simulink model "foc_controller"  (R2023b)
settings: Solver=FixedStepDiscrete  StartTime=0.0  StopTime=0.01  FixedStep=Ts_ctrl  RelTol=1e-3
model workspace (MATLAB code in the model file):
  | % FOC controller parameters
  | % Placeholder values for structural modelling only; no tuning intended.
  | 
  | fs_ctrl = 5000.0;    % controller discrete update frequency [Hz] (placeholder)
  | Ts_ctrl = 1/fs_ctrl; % controller discrete update period [s] (placeholder)
  | 
  | Kp_id = 5;           % d-axis current-loop proportional gain (placeholder)
  | Ki_id = 100;         % d-axis current-loop integral gain (placeholder)
  | 
  | Kp_iq = 5;           % q-axis current-loop proportional gain (placeholder)
  | Ki_iq = 100;         % q-axis current-loop integral gain (placeholder)
  | 
  | Ld_comp = 2e-3;      % d-axis-related compensation coefficient (placeholder)
  | Lq_comp = 2e-3;      % q-axis-related compensation coefficient (placeholder)
  | psi_f_comp = 0.1;    % flux-related compensation coefficient (placeholder)
  | 
  | comp_d_sign = -1;    % d-axis compensation sign (placeholder)
  | comp_q_sign = 1;     % q-axis compensation sign (placeholder)
libraries: slpidlib x2
settings Model: Creator=hwma  LastModifiedBy=hwma

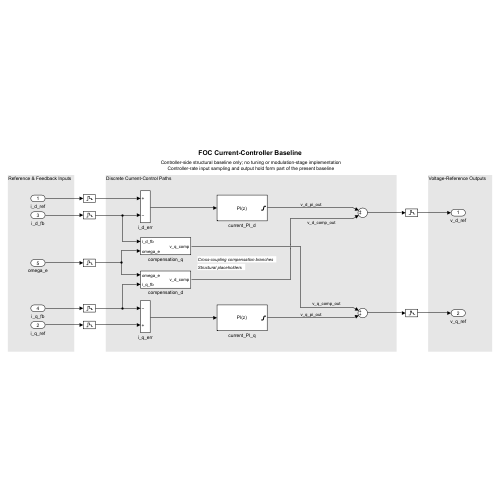
[thumbnail: Simulink's stored preview of the top-level diagram]
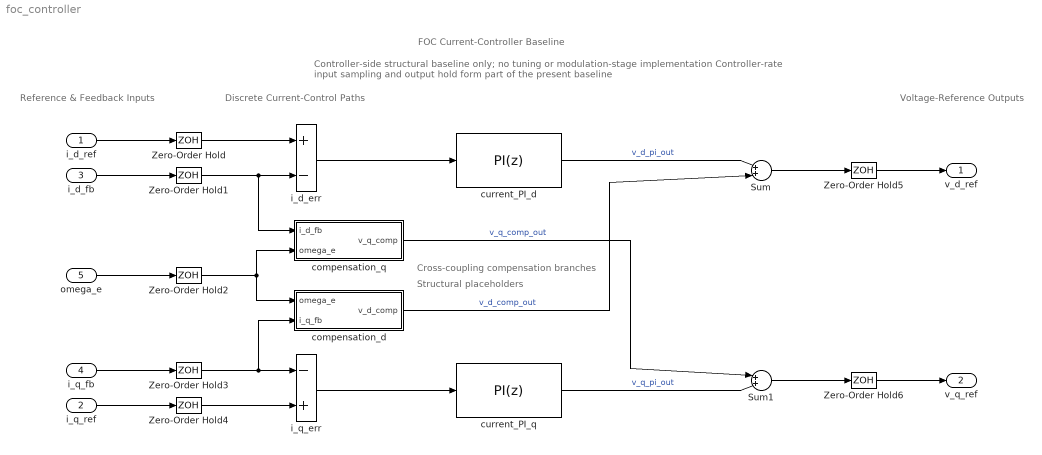
== system foc_controller ==
  note: Cross-coupling compensation branches
  note: Reference & Feedback Inputs
  note: Discrete Current-Control Paths
  note: Voltage-Reference Outputs
  note: Controller-side structural baseline only; no tuning or modulation-stage implementation Controller-rate input sampling and output hold form part of the present baseline
  note: FOC Current-Controller Baseline
  note: Structural placeholders
  i_d_ref : Inport
  i_q_ref : Inport  Port=2
  i_d_fb : Inport  Port=3
  i_q_fb : Inport  Port=4
  omega_e : Inport  Port=5
  Sum : Sum  Inputs=|++|
  Sum1 : Sum  Inputs=|++|
  Zero-Order Hold{,1..6} (7 alike) : ZeroOrderHold  SampleTime=Ts_ctrl
  compensation_d : Subsystem
  compensation_q : Subsystem
  current_PI_d : slpidlib/PID Controller  Controller=PI  Form=Parallel  TimeDomain=Discrete-time  UseExternalTs=off  SampleTime=Ts_ctrl  IntegratorMethod=Forward Euler  FilterMethod=Forward Euler  ControllerParametersSource=internal  P=Kp_id  I=Ki_id  UseKiTs=off  D=0  N=100  UseFilter=on  TunerSelectOption=Transfer Function Based (PID Tuner App)  InitialConditionSource=internal  InitialConditionForIntegrator=0  InitialConditionForFilter=0  DifferentiatorICPrevScaledInput=0  ExternalReset=none  TrackingMode=off  Kt=1  LimitOutput=on  SatLimitsSource=internal  UpperSaturationLimit=440  LowerSaturationLimit=-440  LinearizeAsGain=off  AntiWindupMode=none  Kb=1  LimitIntegrator=on  UpperIntegratorSaturationLimit=440  LowerIntegratorSaturationLimit=-440  POutMin=[]  POutMax=[]  IOutMin=[]  IOutMax=[]  DOutMin=[]  DOutMax=[]  NOutMin=[]  NOutMax=[]  SumOutMin=[]  SumOutMax=[]  SaturationOutMin=[]  SaturationOutMax=[]  PParamMin=[]  PParamMax=[]  IParamMin=[]  IParamMax=[]  DParamMin=[]  DParamMax=[]  NParamMin=[]  NParamMax=[]  KbParamMin=[]  KbParamMax=[]  KtParamMin=[]  KtParamMax=[]  KbOutMin=[]  KbOutMax=[]  KtOutMin=[]  KtOutMax=[]  IntegratorOutMin=[]  IntegratorOutMax=[]  FilterOutMin=[]  FilterOutMax=[]  SumI1OutMin=[]  SumI1OutMax=[]  SumI2OutMin=[]  SumI2OutMax=[]  SumI3OutMin=[]  SumI3OutMax=[]  SumI4OutMin=[]  SumI4OutMax=[]  SumDOutMin=[]  SumDOutMax=[]  DifferentiatorOutMin=[]  DifferentiatorOutMax=[]  FilterDiffOutCoefMin=[]  FilterDiffOutCoefMax=[]  ReciprocalOutMin=[]  ReciprocalOutMax=[]  SumDenOutMin=[]  SumDenOutMax=[]  SumNumOutMin=[]  SumNumOutMax=[]  DivideOutMin=[]  DivideOutMax=[]  UdiffTsProdOutMin=[]  UdiffTsProdOutMax=[]  NTsProdOutMin=[]  NTsProdOutMax=[]  UintegralTsProdOutMin=[]  UintegralTsProdOutMax=[]  UngainTsProdOutMin=[]  UngainTsProdOutMax=[]  ClampingZeroOutDataTypeStr=Inherit: Inherit via back propagation  ClampingZeroOutMin=[]  ClampingZeroOutMax=[]  FilterDenConstantOutDataTypeStr=Inherit: Inherit via back propagation  FilterDenConstantOutMin=[]  FilterDenConstantOutMax=[]  PCopyOutDataTypeStr=Inherit: Inherit via back propagation  PCopyOutMin=[]  PCopyOutMax=[]  NCopyOutDataTypeStr=Inherit: Inherit via back propagation  NCopyOutMin=[]  NCopyOutMax=[]  IntegratorContinuousStateAttributes=''  IntegratorStateMustResolveToSignalObject=off  IntegratorRTWStateStorageClass=Auto  FilterContinuousStateAttributes=''  FilterStateMustResolveToSignalObject=off  FilterRTWStateStorageClass=Auto  ParallelPVariant=InternalParameters  IdealPVariant=Disabled  IVariant=InternalParameters  DVariant=Disabled  IntegratorVariant=Discrete  SatVariant=Enabled  AWVariant=Passthrough  PCopyVariant=Disabled  TRVariant=Disabled  FdbkBlocksVariant=Forward  IdealPFdbkVariant=Disabled  SatFdbkVariant=Disabled  DerivativeFilterVariant=Disabled  NVariant=Disabled  NCopyVariant=Disabled_SignalSpec  FilterICVariant=Disabled  IntegratorICVariant=InternalICs  ExternalResetVariant=Disabled  TRSumVariant=Passthrough  SumFdbkVariant=Disabled  SumVariant=Sum_PI  TsampFilterVariant=InternalTs  TsampNgainVariant=Passthrough  TsampIntegralVariant=Disabled_SignalSpec  ExternalSaturationOutDataTypeStr=Inherit: Same as second input
      settings: LibrarySourceBlock=simulink/Discrete/Discrete PID Controller
  current_PI_q : slpidlib/PID Controller  Controller=PI  Form=Parallel  TimeDomain=Discrete-time  UseExternalTs=off  SampleTime=Ts_ctrl  IntegratorMethod=Forward Euler  FilterMethod=Forward Euler  ControllerParametersSource=internal  P=Kp_iq  I=Ki_iq  UseKiTs=off  D=0  N=100  UseFilter=on  TunerSelectOption=Transfer Function Based (PID Tuner App)  InitialConditionSource=internal  InitialConditionForIntegrator=0  InitialConditionForFilter=0  DifferentiatorICPrevScaledInput=0  ExternalReset=none  TrackingMode=off  Kt=1  LimitOutput=on  SatLimitsSource=internal  UpperSaturationLimit=440  LowerSaturationLimit=-440  LinearizeAsGain=off  AntiWindupMode=none  Kb=1  LimitIntegrator=on  UpperIntegratorSaturationLimit=440  LowerIntegratorSaturationLimit=-440  POutMin=[]  POutMax=[]  IOutMin=[]  IOutMax=[]  DOutMin=[]  DOutMax=[]  NOutMin=[]  NOutMax=[]  SumOutMin=[]  SumOutMax=[]  SaturationOutMin=[]  SaturationOutMax=[]  PParamMin=[]  PParamMax=[]  IParamMin=[]  IParamMax=[]  DParamMin=[]  DParamMax=[]  NParamMin=[]  NParamMax=[]  KbParamMin=[]  KbParamMax=[]  KtParamMin=[]  KtParamMax=[]  KbOutMin=[]  KbOutMax=[]  KtOutMin=[]  KtOutMax=[]  IntegratorOutMin=[]  IntegratorOutMax=[]  FilterOutMin=[]  FilterOutMax=[]  SumI1OutMin=[]  SumI1OutMax=[]  SumI2OutMin=[]  SumI2OutMax=[]  SumI3OutMin=[]  SumI3OutMax=[]  SumI4OutMin=[]  SumI4OutMax=[]  SumDOutMin=[]  SumDOutMax=[]  DifferentiatorOutMin=[]  DifferentiatorOutMax=[]  FilterDiffOutCoefMin=[]  FilterDiffOutCoefMax=[]  ReciprocalOutMin=[]  ReciprocalOutMax=[]  SumDenOutMin=[]  SumDenOutMax=[]  SumNumOutMin=[]  SumNumOutMax=[]  DivideOutMin=[]  DivideOutMax=[]  UdiffTsProdOutMin=[]  UdiffTsProdOutMax=[]  NTsProdOutMin=[]  NTsProdOutMax=[]  UintegralTsProdOutMin=[]  UintegralTsProdOutMax=[]  UngainTsProdOutMin=[]  UngainTsProdOutMax=[]  ClampingZeroOutDataTypeStr=Inherit: Inherit via back propagation  ClampingZeroOutMin=[]  ClampingZeroOutMax=[]  FilterDenConstantOutDataTypeStr=Inherit: Inherit via back propagation  FilterDenConstantOutMin=[]  FilterDenConstantOutMax=[]  PCopyOutDataTypeStr=Inherit: Inherit via back propagation  PCopyOutMin=[]  PCopyOutMax=[]  NCopyOutDataTypeStr=Inherit: Inherit via back propagation  NCopyOutMin=[]  NCopyOutMax=[]  IntegratorContinuousStateAttributes=''  IntegratorStateMustResolveToSignalObject=off  IntegratorRTWStateStorageClass=Auto  FilterContinuousStateAttributes=''  FilterStateMustResolveToSignalObject=off  FilterRTWStateStorageClass=Auto  ParallelPVariant=InternalParameters  IdealPVariant=Disabled  IVariant=InternalParameters  DVariant=Disabled  IntegratorVariant=Discrete  SatVariant=Enabled  AWVariant=Passthrough  PCopyVariant=Disabled  TRVariant=Disabled  FdbkBlocksVariant=Forward  IdealPFdbkVariant=Disabled  SatFdbkVariant=Disabled  DerivativeFilterVariant=Disabled  NVariant=Disabled  NCopyVariant=Disabled_SignalSpec  FilterICVariant=Disabled  IntegratorICVariant=InternalICs  ExternalResetVariant=Disabled  TRSumVariant=Passthrough  SumFdbkVariant=Disabled  SumVariant=Sum_PI  TsampFilterVariant=InternalTs  TsampNgainVariant=Passthrough  TsampIntegralVariant=Disabled_SignalSpec  ExternalSaturationOutDataTypeStr=Inherit: Same as second input
      settings: LibrarySourceBlock=simulink/Discrete/Discrete PID Controller
  i_d_err : Sum  Inputs=+-
  i_q_err : Sum  Inputs=-+
  v_d_ref : Outport
  v_q_ref : Outport  Port=2
  wires:
  i_d_ref/1 -> Zero-Order Hold/1
  i_d_fb/1 -> Zero-Order Hold1/1
  i_q_err/1 -> current_PI_q/1
  current_PI_d/1 -> Sum/1  "v_d_pi_out"
  compensation_d/1(v_d_comp) -> Sum/2  "v_d_comp_out"
  Sum/1 -> Zero-Order Hold5/1
  Sum1/1 -> Zero-Order Hold6/1
  i_d_err/1 -> current_PI_d/1
  current_PI_q/1 -> Sum1/2  "v_q_pi_out"
  compensation_q/1(v_q_comp) -> Sum1/1  "v_q_comp_out"
  omega_e/1 -> Zero-Order Hold2/1
  i_q_fb/1 -> Zero-Order Hold3/1
  i_q_ref/1 -> Zero-Order Hold4/1
  Zero-Order Hold/1 -> i_d_err/1
  Zero-Order Hold1/1 -> compensation_q/1(i_d_fb), i_d_err/2
  Zero-Order Hold2/1 -> compensation_d/1(omega_e), compensation_q/2(omega_e)
  Zero-Order Hold3/1 -> compensation_d/2(i_q_fb), i_q_err/1
  Zero-Order Hold4/1 -> i_q_err/2
  Zero-Order Hold5/1 -> v_d_ref/1
  Zero-Order Hold6/1 -> v_q_ref/1

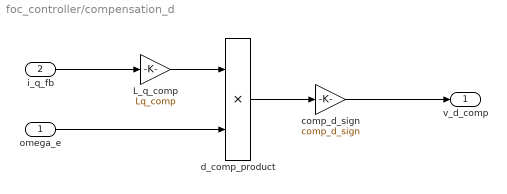
== system foc_controller/compensation_d ==
  omega_e : Inport
  i_q_fb : Inport  Port=2
  L_q_comp : Gain  Gain=Lq_comp
  comp_d_sign : Gain  Gain=comp_d_sign
  d_comp_product : Product
  v_d_comp : Outport
  wires:
  L_q_comp/1 -> d_comp_product/1
  omega_e/1 -> d_comp_product/2
  i_q_fb/1 -> L_q_comp/1
  d_comp_product/1 -> comp_d_sign/1
  comp_d_sign/1 -> v_d_comp/1

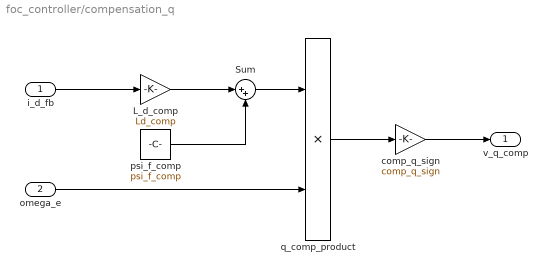
== system foc_controller/compensation_q ==
  i_d_fb : Inport
  omega_e : Inport  Port=2
  L_d_comp : Gain  Gain=Ld_comp
  Sum : Sum  Inputs=|++
  comp_q_sign : Gain  Gain=comp_q_sign
  psi_f_comp : Constant  Value=psi_f_comp
  q_comp_product : Product
  v_q_comp : Outport
  wires:
  i_d_fb/1 -> L_d_comp/1
  L_d_comp/1 -> Sum/1
  psi_f_comp/1 -> Sum/2
  Sum/1 -> q_comp_product/1
  omega_e/1 -> q_comp_product/2
  q_comp_product/1 -> comp_q_sign/1
  comp_q_sign/1 -> v_q_comp/1
